simulink model "test_model"  (R2019b)
settings: Solver=FixedStepAuto  StartTime=0.0  StopTime=10.0  RelTol=1e-3
settings Model: Creator=georgnestlinger  LastModifiedBy=Georg
settings DebuggingCC: ArithmeticOperatorsInVariantConditions=warning
settings SFSimCC: CustomCodeUndefinedFunction=UseInterfaceOnly

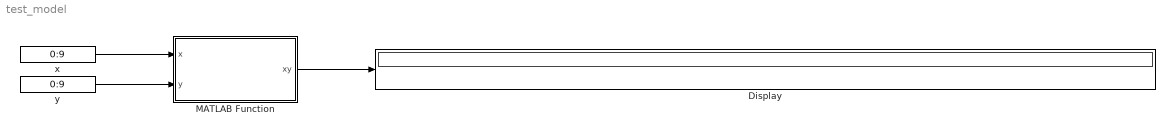
== system test_model ==
  Display : Display
  MATLAB Function : MATLAB Function  TreatAsAtomicUnit=on
  x : Constant  Value=0:9
  y : Constant  Value=0:9
  wires:
  x/1 -> MATLAB Function/1(x)
  y/1 -> MATLAB Function/2(y)
  MATLAB Function/1(xy) -> Display/1

== matlab function test_model/MATLAB Function ==
  data: x input; xy output size=[2, 1e3]; y input
function xy = WaypointsTest(x, y)
coder.extrinsic('warning')

p = Waypoints.xy2Waypoints(x, y);
p = rotate(p, pi/4);
p = p.resample(.5);

xy = [p.x, p.y]';

end%fcn
